simulink model "chris_3R_hsv_mag"  (R2024b)
settings: Solver=FixedStepDiscrete  StartTime=0.0  StopTime=6  FixedStep=0.1  MaxStep=0.1  RelTol=1e-3
libraries: realtime_pacer_lib x1
(part 1 of 2)
settings Model: Creator=RSL  LastModifiedBy=cwaight
settings SolverCC: AlgebraicLoopSolver=TrustRegion
settings DataIOCC: ReturnWorkspaceOutputs=off
settings DebuggingCC: UnconnectedInputMsg=warning  UnconnectedOutputMsg=warning  UnconnectedLineMsg=warning  ArithmeticOperatorsInVariantConditions=warning
settings ModelReferenceCC: EnableRefExpFcnMdlSchedulingChecks=on
settings SFSimCC: SimUseLocalCustomCode=off  CustomCodeUndefinedFunction=UseInterfaceOnly
settings RTWCC: RTWUseLocalCustomCode=off  GPUComputeCapability=3.5
settings CodeAppCC: StateflowObjectComments=on

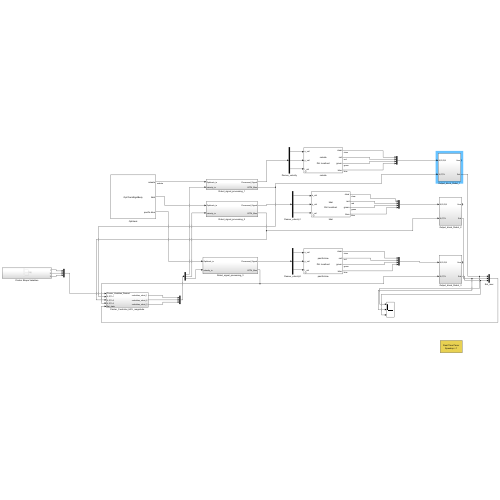
[thumbnail: Simulink's stored preview of the top-level diagram]
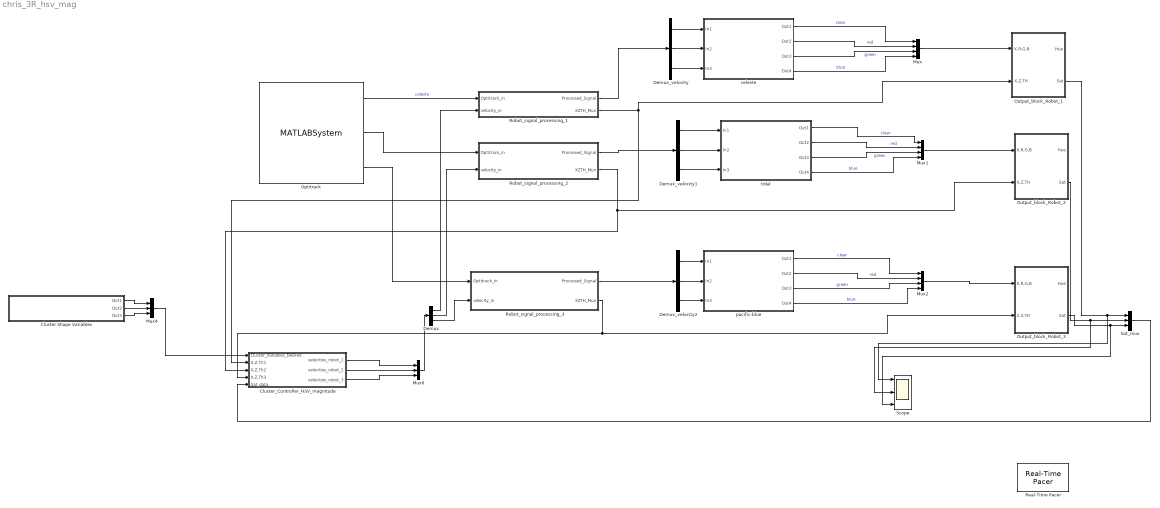
== system chris_3R_hsv_mag ==
  Cluster Shape Variables : Subsystem
  Cluster_Controller_HSV_magnitude : Subsystem
  Demux : Demux  Outputs=3
  Demux_velocity : Demux  Outputs=3
  Demux_velocity1 : Demux  Outputs=3
  Demux_velocity2 : Demux  Outputs=3
  Mux : Mux
  Mux1 : Mux
  Mux2 : Mux
  Mux4 : Mux  Inputs=3
  Mux6 : Mux  Inputs=3
  Optitrack : MATLABSystem  System=OptiTrackRigidBody  coordinateTransformationMatrix=[ 1, 0, 0; 0, 0, 1; 0, -1, 0 ]  rigidBodyNames={ 'celeste','tidal','pacific-blue'}  orientationFormat=Euler angles  debug=on  natNetHostAddress=127.0.0.1  natNetClientAddress=127.0.0.1  dllPath=C:\DecaMATLAB\NatNetSDK\lib\x64\NatNetML.dll  unicast=off
      mask Type: OptiTrackRigidBody
      mask Display:
      | disp('OptiTrackRigidBody');
      | port_label('output',1,'celeste');
      | port_label('output',2,'tidal');
      | port_label('output',3,'pacific-blue');
  Output_block_Robot_1 : Subsystem
  Output_block_Robot_2 : Subsystem
  Output_block_Robot_3 : Subsystem
  Real-Time Pacer : realtime_pacer_lib/Real-Time Pacer  simTimePerRealTime=1
  Robot_signal_processing_1 : Subsystem
  Robot_signal_processing_2 : Subsystem
  Robot_signal_processing_3 : Subsystem
  Sat_mux : Mux  Inputs=3
  Scope : Scope  NumInputPorts=3
  celeste : Subsystem  mask(DecabotMask){robotName=celeste, decabotHelper=localhost, robotAddress=, useDataTurbine=off, useDirectSocket=on, debug=off}
      mask prompts: robotName "Robot name:"; decabotHelper "DecabotHelper/DataTurbine server:"; robotAddress "Robot network address (optional):"; useDataTurbine "Use DataTurbine"; useDirectSocket "Use direct robot TCP connection"; debug "Log debug messages"
      mask help: This is a masked subsystem that contains a Decabot block for bidirectional communication with a decabot over a direct TCP socket connection.
      mask init:
      | robotName = 'Nobody';
      | decabotHelper = 'localhost';
      | robotAddress = '';
      | useDataTurbine = true;
      | debug = true;
      mask TypeOptions robotName: decabot/robotName
      mask Callback robotName:
      | try
      |     set_param( gcb( ), 'Name', get_param( gcb( ), 'robotName' ) );
      | end
      mask TypeOptions decabotHelper: decabot/decabotHelper
      mask TypeOptions robotAddress: decabot/robotAddress
      mask TypeOptions useDataTurbine: decabot/useDataTurbine
      mask TypeOptions useDirectSocket: decabot/useDirectSocket
      mask TypeOptions debug: decabot/debug
      mask Display:
      | disp( [get_param( gcb( ), 'robotName' ) '\n\nDH: ' get_param( gcb( ), 'decabotHelper' ) ] );
      | 
      | port_label('input',1,'x_vel');
      | port_label('input',2,'y_vel');
      | port_label('input',3,'t_vel');
      | 
      | port_label('output',1,'clear');
      | port_label('output',2,'red');
      | port_label('output',3,'green');
      | port_label('output',4,'blue');
  pacific-blue : Subsystem  mask(DecabotMask){robotName=pacific-blue, decabotHelper=localhost, robotAddress=, useDataTurbine=off, useDirectSocket=on, debug=off}
      mask prompts: robotName "Robot name:"; decabotHelper "DecabotHelper/DataTurbine server:"; robotAddress "Robot network address (optional):"; useDataTurbine "Use DataTurbine"; useDirectSocket "Use direct robot TCP connection"; debug "Log debug messages"
      mask help: This is a masked subsystem that contains a Decabot block for bidirectional communication with a decabot over a direct TCP socket connection.
      mask init:
      | robotName = 'Nobody';
      | decabotHelper = 'localhost';
      | robotAddress = '';
      | useDataTurbine = true;
      | debug = true;
      mask TypeOptions robotName: decabot/robotName
      mask Callback robotName:
      | try
      |     set_param( gcb( ), 'Name', get_param( gcb( ), 'robotName' ) );
      | end
      mask TypeOptions decabotHelper: decabot/decabotHelper
      mask TypeOptions robotAddress: decabot/robotAddress
      mask TypeOptions useDataTurbine: decabot/useDataTurbine
      mask TypeOptions useDirectSocket: decabot/useDirectSocket
      mask TypeOptions debug: decabot/debug
      mask Display:
      | disp( [get_param( gcb( ), 'robotName' ) '\n\nDH: ' get_param( gcb( ), 'decabotHelper' ) ] );
      | 
      | port_label('input',1,'x_vel');
      | port_label('input',2,'y_vel');
      | port_label('input',3,'t_vel');
      | 
      | port_label('output',1,'clear');
      | port_label('output',2,'red');
      | port_label('output',3,'green');
      | port_label('output',4,'blue');
  tidal : Subsystem  mask(DecabotMask){robotName=tidal, decabotHelper=localhost, robotAddress=, useDataTurbine=off, useDirectSocket=on, debug=off}
      mask prompts: robotName "Robot name:"; decabotHelper "DecabotHelper/DataTurbine server:"; robotAddress "Robot network address (optional):"; useDataTurbine "Use DataTurbine"; useDirectSocket "Use direct robot TCP connection"; debug "Log debug messages"
      mask help: This is a masked subsystem that contains a Decabot block for bidirectional communication with a decabot over a direct TCP socket connection.
      mask init:
      | robotName = 'Nobody';
      | decabotHelper = 'localhost';
      | robotAddress = '';
      | useDataTurbine = true;
      | debug = true;
      mask TypeOptions robotName: decabot/robotName
      mask Callback robotName:
      | try
      |     set_param( gcb( ), 'Name', get_param( gcb( ), 'robotName' ) );
      | end
      mask TypeOptions decabotHelper: decabot/decabotHelper
      mask TypeOptions robotAddress: decabot/robotAddress
      mask TypeOptions useDataTurbine: decabot/useDataTurbine
      mask TypeOptions useDirectSocket: decabot/useDirectSocket
      mask TypeOptions debug: decabot/debug
      mask Display:
      | disp( [get_param( gcb( ), 'robotName' ) '\n\nDH: ' get_param( gcb( ), 'decabotHelper' ) ] );
      | 
      | port_label('input',1,'x_vel');
      | port_label('input',2,'y_vel');
      | port_label('input',3,'t_vel');
      | 
      | port_label('output',1,'clear');
      | port_label('output',2,'red');
      | port_label('output',3,'green');
      | port_label('output',4,'blue');
  wires:
  Demux_velocity/3 -> celeste/3(In3)
  Demux_velocity/1 -> celeste/1(In1)
  Demux_velocity/2 -> celeste/2(In2)
  Optitrack/1 -> Robot_signal_processing_1/1(Optitrack_in)  "celeste"
  Robot_signal_processing_1/1(Processed_Signal) -> Demux_velocity/1
  celeste/1(Out1) -> Mux/1  "clear"
  celeste/2(Out2) -> Mux/2  "red"
  celeste/3(Out3) -> Mux/3  "green"
  celeste/4(Out4) -> Mux/4  "blue"
  Robot_signal_processing_1/2(XZTH_Mux) -> Output_block_Robot_1/2(X,Z,TH), Cluster_Controller_HSV_magnitude/2(X,Z,Th1)
  Mux/1 -> Output_block_Robot_1/1(K,R,G,B)
  Demux_velocity1/3 -> tidal/3(In3)
  Demux_velocity1/1 -> tidal/1(In1)
  Demux_velocity1/2 -> tidal/2(In2)
  Robot_signal_processing_2/1(Processed_Signal) -> Demux_velocity1/1
  tidal/1(Out1) -> Mux1/1  "clear"
  tidal/2(Out2) -> Mux1/2  "red"
  tidal/3(Out3) -> Mux1/3  "green"
  tidal/4(Out4) -> Mux1/4  "blue"
  Mux1/1 -> Output_block_Robot_2/1(K,R,G,B)
  Demux_velocity2/3 -> pacific-blue/3(In3)
  Demux_velocity2/1 -> pacific-blue/1(In1)
  Demux_velocity2/2 -> pacific-blue/2(In2)
  Robot_signal_processing_3/1(Processed_Signal) -> Demux_velocity2/1
  pacific-blue/1(Out1) -> Mux2/1  "clear"
  pacific-blue/2(Out2) -> Mux2/2  "red"
  pacific-blue/3(Out3) -> Mux2/3  "green"
  pacific-blue/4(Out4) -> Mux2/4  "blue"
  Mux2/1 -> Output_block_Robot_3/1(K,R,G,B)
  Robot_signal_processing_3/2(XZTH_Mux) -> Output_block_Robot_3/2(X,Z,TH), Cluster_Controller_HSV_magnitude/4(X,Z,Th3)
  Optitrack/2 -> Robot_signal_processing_2/1(Optitrack_in)
  Optitrack/3 -> Robot_signal_processing_3/1(Optitrack_in)
  Mux4/1 -> Cluster_Controller_HSV_magnitude/1(Cluster_Variables_Desired)
  Robot_signal_processing_2/2(XZTH_Mux) -> Output_block_Robot_2/2(X,Z,TH), Cluster_Controller_HSV_magnitude/3(X,Z,Th2)
  Cluster Shape Variables/1(Out1) -> Mux4/1
  Cluster Shape Variables/2(Out2) -> Mux4/2
  Cluster Shape Variables/3(Out3) -> Mux4/3
  Demux/1 -> Robot_signal_processing_1/2(velocity_in)
  Demux/2 -> Robot_signal_processing_2/2(velocity_in)
  Demux/3 -> Robot_signal_processing_3/2(velocity_in)
  Mux6/1 -> Demux/1
  Output_block_Robot_1/2(Sat) -> Scope/1, Sat_mux/1
  Output_block_Robot_3/2(Sat) -> Scope/3, Sat_mux/3
  Output_block_Robot_2/2(Sat) -> Scope/2, Sat_mux/2
  Sat_mux/1 -> Cluster_Controller_HSV_magnitude/5(Sat_data)
  Cluster_Controller_HSV_magnitude/1(velocities_robot_1) -> Mux6/1
  Cluster_Controller_HSV_magnitude/2(velocities_robot_2) -> Mux6/2
  Cluster_Controller_HSV_magnitude/3(velocities_robot_3) -> Mux6/3

== system chris_3R_hsv_mag/Cluster Shape Variables ==
  Cluster Variable C : Constant  Value=pi/3
  Cluster_Variable_B : Constant  Value=0.28
  Cluster_variable_A : Constant  Value=0.28
  Out1 : Outport
  Out2 : Outport  Port=2
  Out3 : Outport  Port=3
  wires:
  Cluster_variable_A/1 -> Out1/1
  Cluster Variable C/1 -> Out3/1
  Cluster_Variable_B/1 -> Out2/1

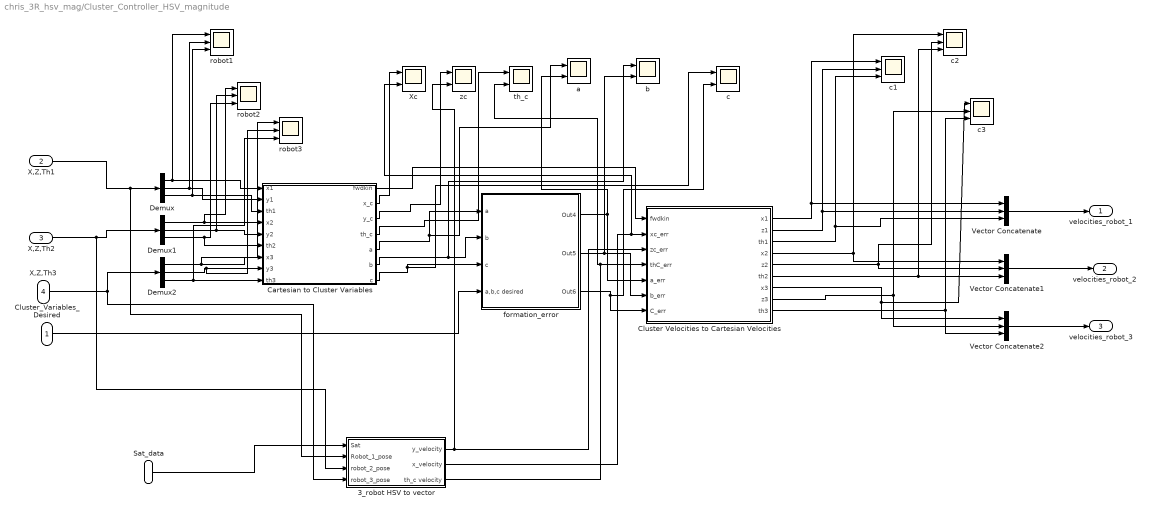
== system chris_3R_hsv_mag/Cluster_Controller_HSV_magnitude ==
  Cluster_Variables_Desired : Inport
  X,Z,Th1 : Inport  Port=2
  X,Z,Th2 : Inport  Port=3
  X,Z,Th3 : Inport  Port=4
  Sat_data : Inport  Port=5
  3_robot HSV to vector : Subsystem
  Cartesian to Cluster Variables : MATLAB Function  TreatAsAtomicUnit=on
  Cluster Velocities to Cartesian Velocities : MATLAB Function  TreatAsAtomicUnit=on
  Demux : Demux  Outputs=3
  Demux1 : Demux  Outputs=3
  Demux2 : Demux  Outputs=3
  Vector Concatenate : Concatenate  NumInputs=3
  Vector Concatenate1 : Concatenate  NumInputs=3
  Vector Concatenate2 : Concatenate  NumInputs=3
  Xc : Scope  NumInputPorts=2
  a : Scope  NumInputPorts=2
  b : Scope  NumInputPorts=2
  c : Scope  NumInputPorts=2
  c1 : Scope  NumInputPorts=3
  c2 : Scope  NumInputPorts=3
  c3 : Scope  NumInputPorts=3
  formation_error : Subsystem
  robot1 : Scope  NumInputPorts=3
  robot2 : Scope  NumInputPorts=3
  robot3 : Scope  NumInputPorts=3
  th_c : Scope  NumInputPorts=2
  zc : Scope  NumInputPorts=2
  velocities_robot_1 : Outport
  velocities_robot_2 : Outport  Port=2
  velocities_robot_3 : Outport  Port=3
  wires:
  X,Z,Th1/1 -> 3_robot HSV to vector/2(Robot_1_pose), Demux/1
  X,Z,Th2/1 -> 3_robot HSV to vector/3(robot_2_pose), Demux1/1
  X,Z,Th3/1 -> Demux2/1, 3_robot HSV to vector/4(robot_3_pose)
  Vector Concatenate/1 -> velocities_robot_1/1
  Cluster Velocities to Cartesian Velocities/2(z1) -> c1/2, Vector Concatenate/2
  Cluster Velocities to Cartesian Velocities/1(x1) -> c1/1, Vector Concatenate/1
  Vector Concatenate1/1 -> velocities_robot_2/1
  Cluster Velocities to Cartesian Velocities/5(z2) -> c2/2, Vector Concatenate1/2
  Cluster Velocities to Cartesian Velocities/4(x2) -> c2/1, Vector Concatenate1/1
  Vector Concatenate2/1 -> velocities_robot_3/1
  Cluster Velocities to Cartesian Velocities/8(z3) -> c3/2, Vector Concatenate2/2
  Cluster Velocities to Cartesian Velocities/7(x3) -> Vector Concatenate2/1, c3/1
  Demux/1 -> robot1/1, Cartesian to Cluster Variables/1(x1)
  Demux/2 -> robot1/2, Cartesian to Cluster Variables/2(y1)
  Demux/3 -> robot1/3, Cartesian to Cluster Variables/3(th1)
  Demux1/1 -> robot2/1, Cartesian to Cluster Variables/4(x2)
  Demux1/2 -> robot2/2, Cartesian to Cluster Variables/5(y2)
  Demux1/3 -> robot2/3, Cartesian to Cluster Variables/6(th2)
  Demux2/1 -> robot3/1, Cartesian to Cluster Variables/7(x3)
  Demux2/2 -> robot3/2, Cartesian to Cluster Variables/8(y3)
  Demux2/3 -> robot3/3, Cartesian to Cluster Variables/9(th3)
  Cartesian to Cluster Variables/2(x_c) -> Xc/1
  Cartesian to Cluster Variables/3(y_c) -> zc/1
  Cartesian to Cluster Variables/4(th_c) -> th_c/1
  Cartesian to Cluster Variables/5(a) -> a/1, formation_error/1(a)
  Cartesian to Cluster Variables/6(b) -> b/1, formation_error/2(b)
  Cartesian to Cluster Variables/7(c) -> c/1, formation_error/3(c)
  Cluster_Variables_Desired/1 -> formation_error/4(a,b,c desired)
  formation_error/1(Out4) -> a/2, Cluster Velocities to Cartesian Velocities/5(a_err)
  formation_error/2(Out5) -> b/2, Cluster Velocities to Cartesian Velocities/6(b_err)
  formation_error/3(Out6) -> Cluster Velocities to Cartesian Velocities/7(C_err), c/2
  Cartesian to Cluster Variables/1(fwdkin) -> Cluster Velocities to Cartesian Velocities/1(fwdkin)
  Cluster Velocities to Cartesian Velocities/3(th1) -> c1/3, Vector Concatenate/3
  Cluster Velocities to Cartesian Velocities/6(th2) -> c2/3, Vector Concatenate1/3
  Cluster Velocities to Cartesian Velocities/9(th3) -> c3/3, Vector Concatenate2/3
  Sat_data/1 -> 3_robot HSV to vector/1(Sat)
  3_robot HSV to vector/2(x_velocity) -> Xc/2, Cluster Velocities to Cartesian Velocities/2(xc_err)
  3_robot HSV to vector/1(y_velocity) -> Cluster Velocities to Cartesian Velocities/3(zc_err), zc/2
  3_robot HSV to vector/3(th_c velocity) -> Cluster Velocities to Cartesian Velocities/4(thC_err), th_c/2

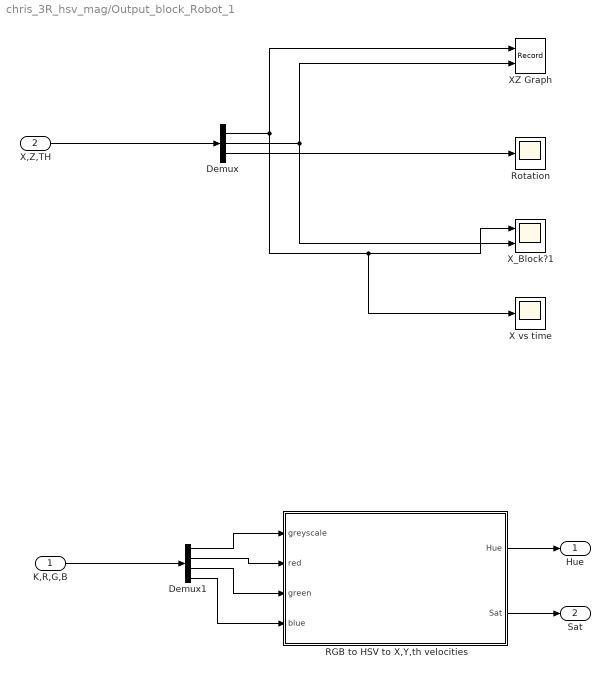
== system chris_3R_hsv_mag/Output_block_Robot_1 ==
  K,R,G,B : Inport
  X,Z,TH : Inport  Port=2
  Demux : Demux  Outputs=3
  Demux1 : Demux
  RGB to HSV to X,Y,th velocities : Subsystem
  Rotation : Scope
  X vs time : Scope
  XZ Graph : Record  FileSettingsInternal="{\"entries\":[{\"content\":{\"excelSettings\":{\"content\":{},\"type\":\"Streamout.ExcelSettings\"}},\"type\":\"Streamout.FileSettingStorage\",\"uuid\":\"\"}],\"packageUris\":[\"http:\\/\\/schema.mathworks.com\\/mf0\\/streamout_blocks\\/R2020a\"],\"version\":\"1.0\"}"  Layout=[1 1]  SignalsInternal="{\"entries\":[{\"content\":{\"signals\":[{\"content\":{\"blockPath\":[],\"dimensions\":[1],\"domain\":\"\",\"lineColor\":\"#fe330a\",\"lineWidth\":2,\"port\":1,\"sid\":[\"\"],\"signalID\":1,\"signalName\":\"Demux:1\"},\"type\":\"RecordBlkView.Signal\",\"uuid\":\"\"},{\"content\":{\"blockPath\":[],\"dimensions\":[1],\"domain\":\"\",\"lineColor\":\"#22b573\",\"lineWidth\":2,\"port\":2,\"sid\":[\"\"],\"signalID\":2,\"signalName\":\"Demux:2\"},\"type\":\"RecordBlkView.Signal\",\"uuid\":\"\"}]},\"type\":\"RecordBlkView.InputSignals\",\"uuid\":\"\"}],\"packageUris\":[\"http:\\/\\/schema.mathworks.com\\/mf0\\/streamout_blocks\\/R2020a\"],\"version\":\"1.0\"}"  VisualizationBindings="{\"xyplotplugin\":{\"info\":[{\"series\":[],\"subplotID\":1}]}}"  CompatibilityTag=XY  st=-1
  X_Block?1 : Scope  NumInputPorts=2
  Hue : Outport
  Sat : Outport  Port=2
  wires:
  Demux/3 -> Rotation/1
  Demux/2 -> X_Block?1/2, XZ Graph/2
  X,Z,TH/1 -> Demux/1
  Demux/1 -> X vs time/1, X_Block?1/1, XZ Graph/1
  K,R,G,B/1 -> Demux1/1
  Demux1/1 -> RGB to HSV to X,Y,th velocities/1(greyscale)
  Demux1/2 -> RGB to HSV to X,Y,th velocities/2(red)
  Demux1/3 -> RGB to HSV to X,Y,th velocities/3(green)
  Demux1/4 -> RGB to HSV to X,Y,th velocities/4(blue)
  RGB to HSV to X,Y,th velocities/1(Hue) -> Hue/1
  RGB to HSV to X,Y,th velocities/2(Sat) -> Sat/1

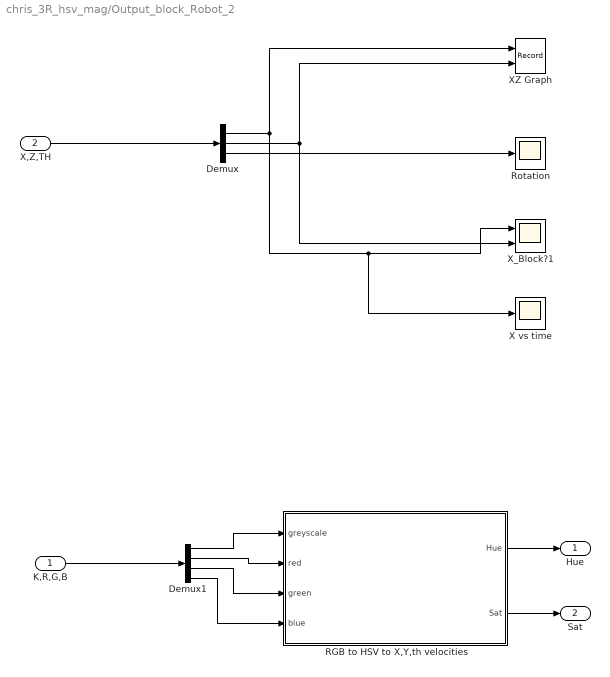
== system chris_3R_hsv_mag/Output_block_Robot_2 ==
  K,R,G,B : Inport
  X,Z,TH : Inport  Port=2
  Demux : Demux  Outputs=3
  Demux1 : Demux
  RGB to HSV to X,Y,th velocities : Subsystem
  Rotation : Scope
  X vs time : Scope
  XZ Graph : Record  FileSettingsInternal="{\"entries\":[{\"content\":{\"excelSettings\":{\"content\":{},\"type\":\"Streamout.ExcelSettings\"}},\"type\":\"Streamout.FileSettingStorage\",\"uuid\":\"\"}],\"packageUris\":[\"http:\\/\\/schema.mathworks.com\\/mf0\\/streamout_blocks\\/R2020a\"],\"version\":\"1.0\"}"  Layout=[1 1]  SignalsInternal="{\"entries\":[{\"content\":{\"signals\":[{\"content\":{\"blockPath\":[],\"dimensions\":[1],\"domain\":\"\",\"lineColor\":\"#edb120\",\"lineWidth\":2,\"port\":1,\"sid\":[\"\"],\"signalID\":1,\"signalName\":\"Demux:1\"},\"type\":\"RecordBlkView.Signal\",\"uuid\":\"\"},{\"content\":{\"blockPath\":[],\"dimensions\":[1],\"domain\":\"\",\"lineColor\":\"#7e2f8e\",\"lineWidth\":2,\"port\":2,\"sid\":[\"\"],\"signalID\":2,\"signalName\":\"Demux:2\"},\"type\":\"RecordBlkView.Signal\",\"uuid\":\"\"}]},\"type\":\"RecordBlkView.InputSignals\",\"uuid\":\"\"}],\"packageUris\":[\"http:\\/\\/schema.mathworks.com\\/mf0\\/streamout_blocks\\/R2020a\"],\"version\":\"1.0\"}"  VisualizationBindings="{\"xyplotplugin\":{\"info\":[{\"series\":[],\"subplotID\":1}]}}"  CompatibilityTag=XY  st=-1
  X_Block?1 : Scope  NumInputPorts=2
  Hue : Outport
  Sat : Outport  Port=2
  wires:
  Demux/3 -> Rotation/1
  Demux/2 -> X_Block?1/2, XZ Graph/2
  X,Z,TH/1 -> Demux/1
  Demux/1 -> X vs time/1, X_Block?1/1, XZ Graph/1
  K,R,G,B/1 -> Demux1/1
  Demux1/1 -> RGB to HSV to X,Y,th velocities/1(greyscale)
  Demux1/2 -> RGB to HSV to X,Y,th velocities/2(red)
  Demux1/3 -> RGB to HSV to X,Y,th velocities/3(green)
  Demux1/4 -> RGB to HSV to X,Y,th velocities/4(blue)
  RGB to HSV to X,Y,th velocities/1(Hue) -> Hue/1
  RGB to HSV to X,Y,th velocities/2(Sat) -> Sat/1

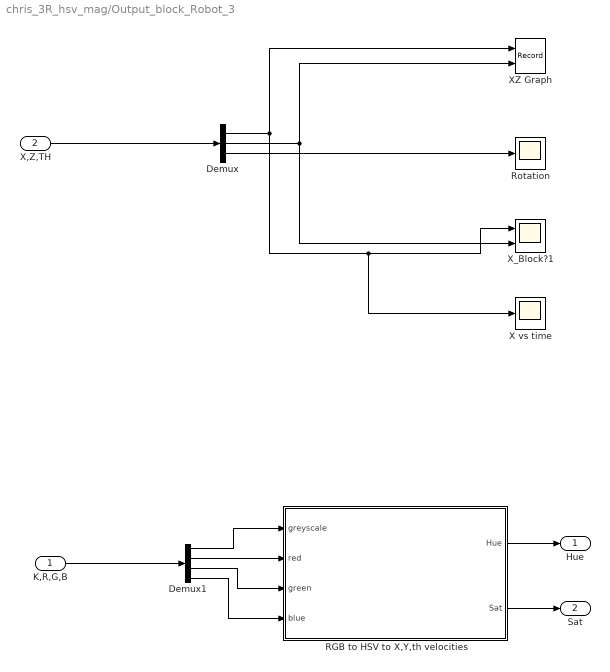
== system chris_3R_hsv_mag/Output_block_Robot_3 ==
  K,R,G,B : Inport
  X,Z,TH : Inport  Port=2
  Demux : Demux  Outputs=3
  Demux1 : Demux
  RGB to HSV to X,Y,th velocities : Subsystem
  Rotation : Scope
  X vs time : Scope
  XZ Graph : Record  FileSettingsInternal="{\"entries\":[{\"content\":{\"excelSettings\":{\"content\":{},\"type\":\"Streamout.ExcelSettings\"}},\"type\":\"Streamout.FileSettingStorage\",\"uuid\":\"\"}],\"packageUris\":[\"http:\\/\\/schema.mathworks.com\\/mf0\\/streamout_blocks\\/R2020a\"],\"version\":\"1.0\"}"  Layout=[1 1]  SignalsInternal="{\"entries\":[{\"content\":{\"signals\":[{\"content\":{\"blockPath\":[],\"dimensions\":[1],\"domain\":\"\",\"lineColor\":\"#a2142f\",\"lineWidth\":2,\"port\":1,\"sid\":[\"\"],\"signalID\":1,\"signalName\":\"Demux:1\"},\"type\":\"RecordBlkView.Signal\",\"uuid\":\"\"},{\"content\":{\"blockPath\":[],\"dimensions\":[1],\"domain\":\"\",\"lineColor\":\"#139fff\",\"lineWidth\":2,\"port\":2,\"sid\":[\"\"],\"signalID\":2,\"signalName\":\"Demux:2\"},\"type\":\"RecordBlkView.Signal\",\"uuid\":\"\"}]},\"type\":\"RecordBlkView.InputSignals\",\"uuid\":\"\"}],\"packageUris\":[\"http:\\/\\/schema.mathworks.com\\/mf0\\/streamout_blocks\\/R2020a\"],\"version\":\"1.0\"}"  VisualizationBindings="{\"xyplotplugin\":{\"info\":[{\"series\":[],\"subplotID\":1}]}}"  CompatibilityTag=XY  st=-1
  X_Block?1 : Scope  NumInputPorts=2
  Hue : Outport
  Sat : Outport  Port=2
  wires:
  Demux/3 -> Rotation/1
  Demux/2 -> X_Block?1/2, XZ Graph/2
  X,Z,TH/1 -> Demux/1
  Demux/1 -> X vs time/1, X_Block?1/1, XZ Graph/1
  K,R,G,B/1 -> Demux1/1
  Demux1/1 -> RGB to HSV to X,Y,th velocities/1(greyscale)
  Demux1/2 -> RGB to HSV to X,Y,th velocities/2(red)
  Demux1/3 -> RGB to HSV to X,Y,th velocities/3(green)
  Demux1/4 -> RGB to HSV to X,Y,th velocities/4(blue)
  RGB to HSV to X,Y,th velocities/1(Hue) -> Hue/1
  RGB to HSV to X,Y,th velocities/2(Sat) -> Sat/1

== system chris_3R_hsv_mag/Robot_signal_processing_1 ==
  Optitrack_in : Inport
  velocity_in : Inport  Port=2
  Demux4 : Demux  Outputs=3
  Global to Body Velocities : Product  Multiplication=Matrix(*)
  Global to Body Rotation Matrix : MATLAB Function  TreatAsAtomicUnit=on
  Math Function : Math  Operator=transpose  SignedPower=on
  Mux : Mux  Inputs=3
  Signal_Reshape : Reshape  OutputDimensions=6
  Signal_Select : Selector  InputPortWidth=6  IndexOptions=Index vector (dialog)  Indices=[1 2 6]  OutputSizes=1
  Processed_Signal : Outport
  XZTH_Mux : Outport  Port=2
  wires:
  Demux4/1 -> Mux/1  "X"
  Demux4/3 -> Mux/3, Global to Body Rotation Matrix/1(u)  "theta"
  Demux4/2 -> Mux/2  "Z"
  Global to Body Velocities/1 -> Processed_Signal/1
  Signal_Reshape/1 -> Signal_Select/1
  velocity_in/1 -> Global to Body Velocities/2
  Optitrack_in/1 -> Signal_Reshape/1
  Global to Body Rotation Matrix/1(y) -> Math Function/1
  Signal_Select/1 -> Demux4/1
  Math Function/1 -> Global to Body Velocities/1
  Mux/1 -> XZTH_Mux/1

== system chris_3R_hsv_mag/Robot_signal_processing_2 ==
  Optitrack_in : Inport
  velocity_in : Inport  Port=2
  Demux4 : Demux  Outputs=3
  Global to Body Velocities : Product  Multiplication=Matrix(*)
  Global to Body Rotation Matrix : MATLAB Function  TreatAsAtomicUnit=on
  Math Function : Math  Operator=transpose  SignedPower=on
  Mux : Mux  Inputs=3
  Signal_Reshape : Reshape  OutputDimensions=6
  Signal_Select : Selector  InputPortWidth=6  IndexOptions=Index vector (dialog)  Indices=[1 2 6]  OutputSizes=1
  Processed_Signal : Outport
  XZTH_Mux : Outport  Port=2
  wires:
  Demux4/1 -> Mux/1  "X"
  Demux4/3 -> Mux/3, Global to Body Rotation Matrix/1(u)  "theta"
  Demux4/2 -> Mux/2  "Z"
  Global to Body Velocities/1 -> Processed_Signal/1
  Signal_Reshape/1 -> Signal_Select/1
  velocity_in/1 -> Global to Body Velocities/2
  Optitrack_in/1 -> Signal_Reshape/1
  Global to Body Rotation Matrix/1(y) -> Math Function/1
  Signal_Select/1 -> Demux4/1
  Math Function/1 -> Global to Body Velocities/1
  Mux/1 -> XZTH_Mux/1

== system chris_3R_hsv_mag/Robot_signal_processing_3 ==
  Optitrack_in : Inport
  velocity_in : Inport  Port=2
  Demux4 : Demux  Outputs=3
  Global to Body Velocities : Product  Multiplication=Matrix(*)
  Global to Body Rotation Matrix : MATLAB Function  TreatAsAtomicUnit=on
  Math Function : Math  Operator=transpose  SignedPower=on
  Mux : Mux  Inputs=3
  Signal_Reshape : Reshape  OutputDimensions=6
  Signal_Select : Selector  InputPortWidth=6  IndexOptions=Index vector (dialog)  Indices=[1 2 6]  OutputSizes=1
  Processed_Signal : Outport
  XZTH_Mux : Outport  Port=2
  wires:
  Demux4/1 -> Mux/1  "X"
  Demux4/3 -> Mux/3, Global to Body Rotation Matrix/1(u)  "theta"
  Demux4/2 -> Mux/2  "Z"
  Global to Body Velocities/1 -> Processed_Signal/1
  Signal_Reshape/1 -> Signal_Select/1
  velocity_in/1 -> Global to Body Velocities/2
  Optitrack_in/1 -> Signal_Reshape/1
  Global to Body Rotation Matrix/1(y) -> Math Function/1
  Signal_Select/1 -> Demux4/1
  Math Function/1 -> Global to Body Velocities/1
  Mux/1 -> XZTH_Mux/1

== system chris_3R_hsv_mag/celeste ==
  In1 : Inport
  In2 : Inport  Port=2
  In3 : Inport  Port=3
  Signal Specification : SignalSpecification  OutDataTypeStr=double  Dimensions=1
  Signal Specification1 : SignalSpecification  OutDataTypeStr=double  Dimensions=1
  Signal Specification2 : SignalSpecification  OutDataTypeStr=double  Dimensions=1
  decabot : MATLABSystem  System=Decabot  robotName=celeste  decabotHelper=localhost  useDataTurbine=off  useDirectSocket=on  debug=off
      mask Type: Decabot
      mask Display:
      | disp('celeste\n\nDH: localhost');
      | port_label('input',1,'x_vel');
      | port_label('input',2,'y_vel');
      | port_label('input',3,'t_vel');
      | port_label('output',1,'clear');
      | port_label('output',2,'red');
      | port_label('output',3,'green');
      | port_label('output',4,'blue');
  Out1 : Outport
  Out2 : Outport  Port=2
  Out3 : Outport  Port=3
  Out4 : Outport  Port=4
  wires:
  Signal Specification2/1 -> decabot/3
  Signal Specification1/1 -> decabot/2
  Signal Specification/1 -> decabot/1
  In2/1 -> Signal Specification1/1
  decabot/4 -> Out4/1
  decabot/1 -> Out1/1
  decabot/3 -> Out3/1
  decabot/2 -> Out2/1
  In1/1 -> Signal Specification/1
  In3/1 -> Signal Specification2/1

== system chris_3R_hsv_mag/pacific-blue ==
  In1 : Inport
  In2 : Inport  Port=2
  In3 : Inport  Port=3
  Signal Specification : SignalSpecification  OutDataTypeStr=double  Dimensions=1
  Signal Specification1 : SignalSpecification  OutDataTypeStr=double  Dimensions=1
  Signal Specification2 : SignalSpecification  OutDataTypeStr=double  Dimensions=1
  decabot : MATLABSystem  System=Decabot  robotName=pacific-blue  decabotHelper=localhost  useDataTurbine=off  useDirectSocket=on  debug=off
      mask Type: Decabot
      mask Display:
      | disp('pacific-blue\n\nDH: localhost');
      | port_label('input',1,'x_vel');
      | port_label('input',2,'y_vel');
      | port_label('input',3,'t_vel');
      | port_label('output',1,'clear');
      | port_label('output',2,'red');
      | port_label('output',3,'green');
      | port_label('output',4,'blue');
  Out1 : Outport
  Out2 : Outport  Port=2
  Out3 : Outport  Port=3
  Out4 : Outport  Port=4
  wires:
  Signal Specification2/1 -> decabot/3
  Signal Specification1/1 -> decabot/2
  Signal Specification/1 -> decabot/1
  In2/1 -> Signal Specification1/1
  decabot/4 -> Out4/1
  decabot/1 -> Out1/1
  decabot/3 -> Out3/1
  decabot/2 -> Out2/1
  In1/1 -> Signal Specification/1
  In3/1 -> Signal Specification2/1

== system chris_3R_hsv_mag/tidal ==
  In1 : Inport
  In2 : Inport  Port=2
  In3 : Inport  Port=3
  Signal Specification : SignalSpecification  OutDataTypeStr=double  Dimensions=1
  Signal Specification1 : SignalSpecification  OutDataTypeStr=double  Dimensions=1
  Signal Specification2 : SignalSpecification  OutDataTypeStr=double  Dimensions=1
  decabot : MATLABSystem  System=Decabot  robotName=tidal  decabotHelper=localhost  useDataTurbine=off  useDirectSocket=on  debug=off
      mask Type: Decabot
      mask Display:
      | disp('tidal\n\nDH: localhost');
      | port_label('input',1,'x_vel');
      | port_label('input',2,'y_vel');
      | port_label('input',3,'t_vel');
      | port_label('output',1,'clear');
      | port_label('output',2,'red');
      | port_label('output',3,'green');
      | port_label('output',4,'blue');
  Out1 : Outport
  Out2 : Outport  Port=2
  Out3 : Outport  Port=3
  Out4 : Outport  Port=4
  wires:
  Signal Specification2/1 -> decabot/3
  Signal Specification1/1 -> decabot/2
  Signal Specification/1 -> decabot/1
  In2/1 -> Signal Specification1/1
  decabot/4 -> Out4/1
  decabot/1 -> Out1/1
  decabot/3 -> Out3/1
  decabot/2 -> Out2/1
  In1/1 -> Signal Specification/1
  In3/1 -> Signal Specification2/1

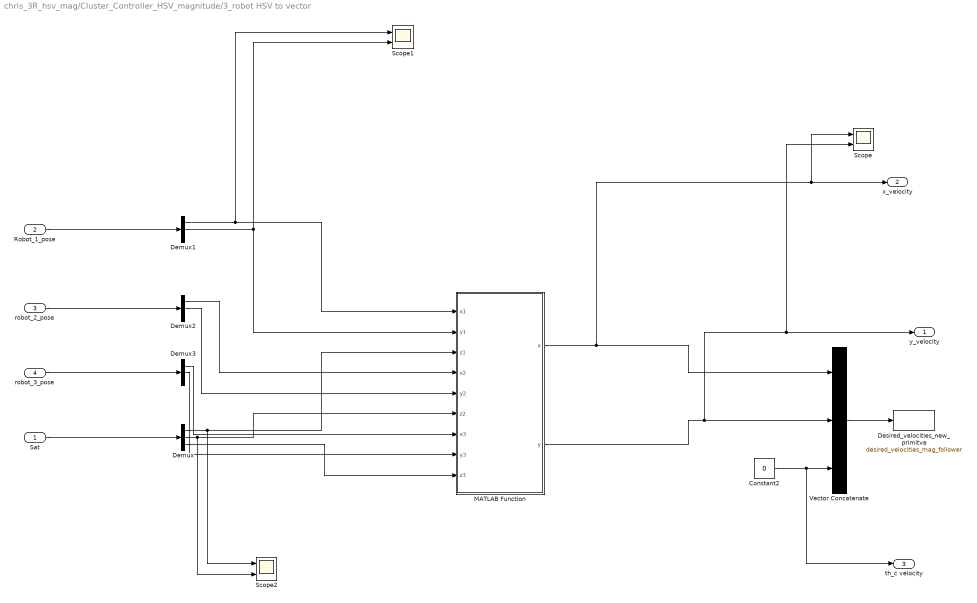
== system chris_3R_hsv_mag/Cluster_Controller_HSV_magnitude/3_robot HSV to vector ==
  Sat : Inport
  Robot_1_pose : Inport  Port=2
  robot_2_pose : Inport  Port=3
  robot_3_pose : Inport  Port=4
  Constant2 : Constant  Value=0
  Demux{,1..3} (4 alike) : Demux  Outputs=3
  Desired_velocities_new_primitve : ToWorkspace  VariableName=desired_velocities_mag_follower  SampleTime=-1
  MATLAB Function : MATLAB Function  TreatAsAtomicUnit=on
  Scope : Scope  NumInputPorts=2
  Scope1 : Scope  NumInputPorts=2
  Scope2 : Scope  NumInputPorts=2
  Vector Concatenate : Concatenate  NumInputs=3
  y_velocity : Outport
  x_velocity : Outport  Port=2
  th_c velocity : Outport  Port=3
  wires:
  Vector Concatenate/1 -> Desired_velocities_new_primitve/1
  Constant2/1 -> th_c velocity/1, Vector Concatenate/3
  Sat/1 -> Demux/1
  Robot_1_pose/1 -> Demux1/1
  robot_2_pose/1 -> Demux2/1
  robot_3_pose/1 -> Demux3/1
  Demux1/1 -> Scope1/1, MATLAB Function/1(x1)
  Demux1/2 -> MATLAB Function/2(y1), Scope1/2
  Demux/1 -> Scope2/1, MATLAB Function/3(z1)
  Demux2/1 -> MATLAB Function/4(x2)
  Demux2/2 -> MATLAB Function/5(y2)
  Demux/2 -> Scope2/2, MATLAB Function/6(z2)
  Demux3/1 -> MATLAB Function/7(x3)
  Demux3/2 -> MATLAB Function/8(y3)
  Demux/3 -> MATLAB Function/9(z3)
  MATLAB Function/1(x) -> Scope/1, x_velocity/1, Vector Concatenate/1
  MATLAB Function/2(y) -> Scope/2, y_velocity/1, Vector Concatenate/2

== system chris_3R_hsv_mag/Cluster_Controller_HSV_magnitude/formation_error ==
  a : Inport
  b : Inport  Port=2
  c : Inport  Port=3
  a,b,c desired : Inport  Port=4
  Demux7 : Demux  Outputs=3
  Sum3 : Sum  Inputs=-+
  Sum4 : Sum  Inputs=-+
  Sum5 : Sum  Inputs=-+
  Out4 : Outport
  Out5 : Outport  Port=2
  Out6 : Outport  Port=3
  wires:
  Sum3/1 -> Out4/1
  Demux7/3 -> Sum5/2
  a,b,c desired/1 -> Demux7/1
  Demux7/1 -> Sum3/2
  b/1 -> Sum4/1
  Demux7/2 -> Sum4/2
  c/1 -> Sum5/1
  Sum4/1 -> Out5/1
  Sum5/1 -> Out6/1
  a/1 -> Sum3/1

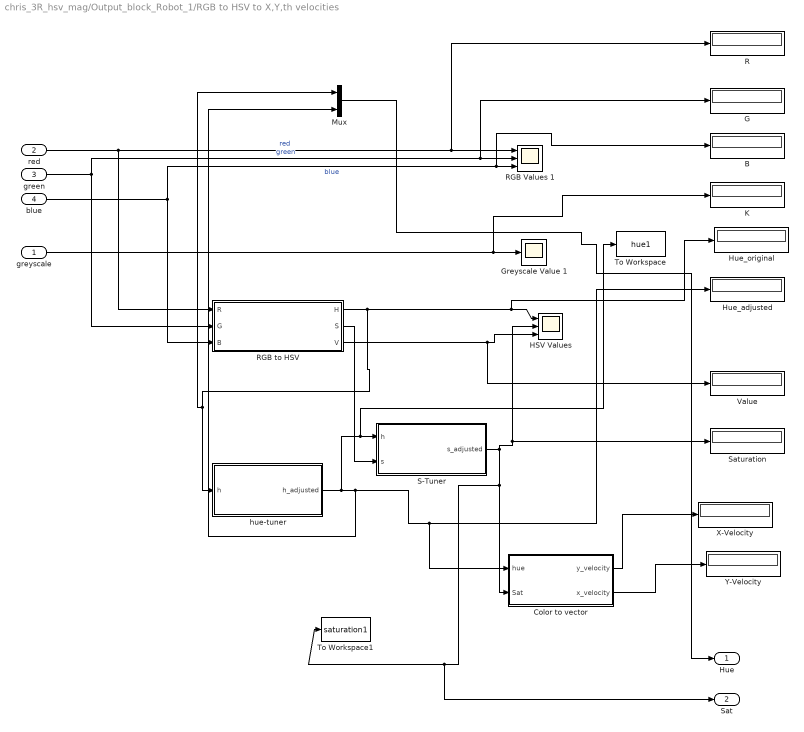
== system chris_3R_hsv_mag/Output_block_Robot_1/RGB to HSV to X,Y,th velocities ==
  greyscale : Inport
  red : Inport  Port=2
  green : Inport  Port=3
  blue : Inport  Port=4
  B : Display
  Color to vector : Subsystem
  G : Display
  Greyscale Value 1 : Scope
  HSV Values : Scope  NumInputPorts=3
  Hue_adjusted : Display
  Hue_original : Display
  K : Display
  Mux : Mux  Inputs=2
  R : Display
  "RGB Values 1 " : Scope  NumInputPorts=3
  RGB to HSV : MATLAB Function  TreatAsAtomicUnit=on
  S-Tuner : MATLAB Function  TreatAsAtomicUnit=on
  Saturation : Display
  To Workspace : ToWorkspace  VariableName=hue1  SaveFormat=Timeseries  SampleTime=-1
  To Workspace1 : ToWorkspace  VariableName=saturation1  SaveFormat=Timeseries  SampleTime=-1
  Value : Display
  X-Velocity : Display
  "Y-Velocity " : Display
  hue-tuner : MATLAB Function  TreatAsAtomicUnit=on
  Hue : Outport
  Sat : Outport  Port=2
  wires:
  red/1 -> R/1, "RGB Values 1 "/1, RGB to HSV/1(R)  "red"
  blue/1 -> B/1, "RGB Values 1 "/3, RGB to HSV/3(B)  "blue"
  greyscale/1 -> K/1, Greyscale Value 1/1
  green/1 -> G/1, "RGB Values 1 "/2, RGB to HSV/2(G)  "green"
  RGB to HSV/3(V) -> Value/1, HSV Values/3
  RGB to HSV/2(S) -> S-Tuner/2(s)
  S-Tuner/1(s_adjusted) -> HSV Values/2, Saturation/1, Sat/1, To Workspace1/1, Color to vector/2(Sat)
  Color to vector/1(y_velocity) -> X-Velocity/1
  Color to vector/2(x_velocity) -> "Y-Velocity "/1
  hue-tuner/1(h_adjusted) -> To Workspace/1, S-Tuner/1(h), Mux/2, Color to vector/1(hue), Hue_adjusted/1
  Mux/1 -> Hue/1
  RGB to HSV/1(H) -> Hue_original/1, HSV Values/1, Mux/1, hue-tuner/1(h)

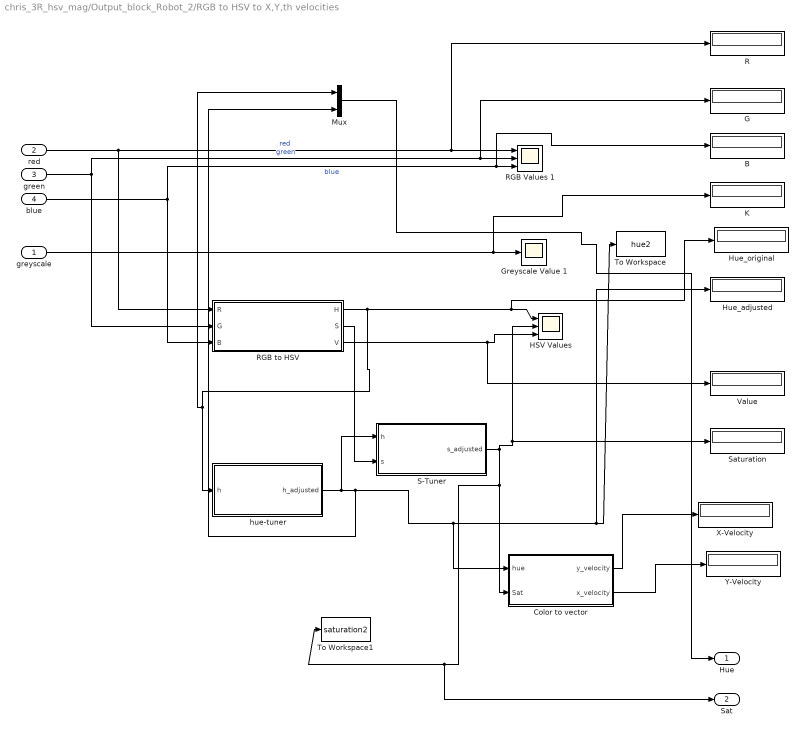
== system chris_3R_hsv_mag/Output_block_Robot_2/RGB to HSV to X,Y,th velocities ==
  greyscale : Inport
  red : Inport  Port=2
  green : Inport  Port=3
  blue : Inport  Port=4
  B : Display
  Color to vector : Subsystem
  G : Display
  Greyscale Value 1 : Scope
  HSV Values : Scope  NumInputPorts=3
  Hue_adjusted : Display
  Hue_original : Display
  K : Display
  Mux : Mux  Inputs=2
  R : Display
  "RGB Values 1 " : Scope  NumInputPorts=3
  RGB to HSV : MATLAB Function  TreatAsAtomicUnit=on
  S-Tuner : MATLAB Function  TreatAsAtomicUnit=on
  Saturation : Display
  To Workspace : ToWorkspace  VariableName=hue2  SaveFormat=Timeseries  SampleTime=-1
  To Workspace1 : ToWorkspace  VariableName=saturation2  SaveFormat=Timeseries  SampleTime=-1
  Value : Display
  X-Velocity : Display
  "Y-Velocity " : Display
  hue-tuner : MATLAB Function  TreatAsAtomicUnit=on
  Hue : Outport
  Sat : Outport  Port=2
  wires:
  red/1 -> R/1, "RGB Values 1 "/1, RGB to HSV/1(R)  "red"
  blue/1 -> B/1, "RGB Values 1 "/3, RGB to HSV/3(B)  "blue"
  greyscale/1 -> K/1, Greyscale Value 1/1
  green/1 -> G/1, "RGB Values 1 "/2, RGB to HSV/2(G)  "green"
  RGB to HSV/3(V) -> Value/1, HSV Values/3
  RGB to HSV/2(S) -> S-Tuner/2(s)
  S-Tuner/1(s_adjusted) -> HSV Values/2, Saturation/1, Sat/1, To Workspace1/1, Color to vector/2(Sat)
  Color to vector/1(y_velocity) -> X-Velocity/1
  Color to vector/2(x_velocity) -> "Y-Velocity "/1
  hue-tuner/1(h_adjusted) -> S-Tuner/1(h), Mux/2, Color to vector/1(hue), To Workspace/1, Hue_adjusted/1
  Mux/1 -> Hue/1
  RGB to HSV/1(H) -> Hue_original/1, HSV Values/1, Mux/1, hue-tuner/1(h)

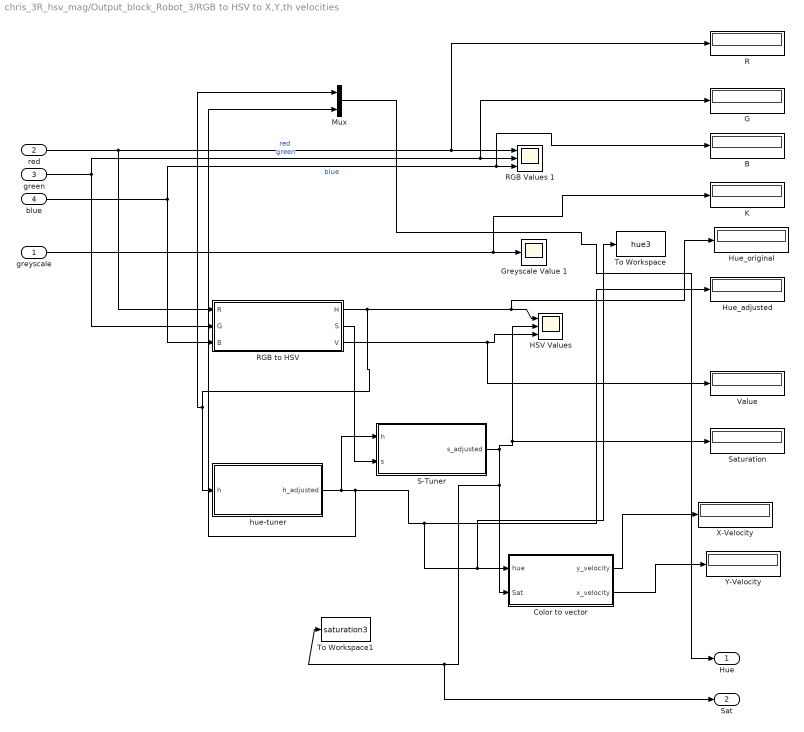
== system chris_3R_hsv_mag/Output_block_Robot_3/RGB to HSV to X,Y,th velocities ==
  greyscale : Inport
  red : Inport  Port=2
  green : Inport  Port=3
  blue : Inport  Port=4
  B : Display
  Color to vector : Subsystem
  G : Display
  Greyscale Value 1 : Scope
  HSV Values : Scope  NumInputPorts=3
  Hue_adjusted : Display
  Hue_original : Display
  K : Display
  Mux : Mux  Inputs=2
  R : Display
  "RGB Values 1 " : Scope  NumInputPorts=3
  RGB to HSV : MATLAB Function  TreatAsAtomicUnit=on
  S-Tuner : MATLAB Function  TreatAsAtomicUnit=on
  Saturation : Display
  To Workspace : ToWorkspace  VariableName=hue3  SaveFormat=Timeseries  SampleTime=-1
  To Workspace1 : ToWorkspace  VariableName=saturation3  SaveFormat=Timeseries  SampleTime=-1
  Value : Display
  X-Velocity : Display
  "Y-Velocity " : Display
  hue-tuner : MATLAB Function  TreatAsAtomicUnit=on
  Hue : Outport
  Sat : Outport  Port=2
  wires:
  red/1 -> R/1, "RGB Values 1 "/1, RGB to HSV/1(R)  "red"
  blue/1 -> B/1, "RGB Values 1 "/3, RGB to HSV/3(B)  "blue"
  greyscale/1 -> K/1, Greyscale Value 1/1
  green/1 -> G/1, "RGB Values 1 "/2, RGB to HSV/2(G)  "green"
  RGB to HSV/3(V) -> Value/1, HSV Values/3
  RGB to HSV/2(S) -> S-Tuner/2(s)
  S-Tuner/1(s_adjusted) -> HSV Values/2, Saturation/1, Sat/1, To Workspace1/1, Color to vector/2(Sat)
  Color to vector/1(y_velocity) -> X-Velocity/1
  Color to vector/2(x_velocity) -> "Y-Velocity "/1
  hue-tuner/1(h_adjusted) -> S-Tuner/1(h), Mux/2, To Workspace/1, Color to vector/1(hue), Hue_adjusted/1
  Mux/1 -> Hue/1
  RGB to HSV/1(H) -> Hue_original/1, HSV Values/1, Mux/1, hue-tuner/1(h)

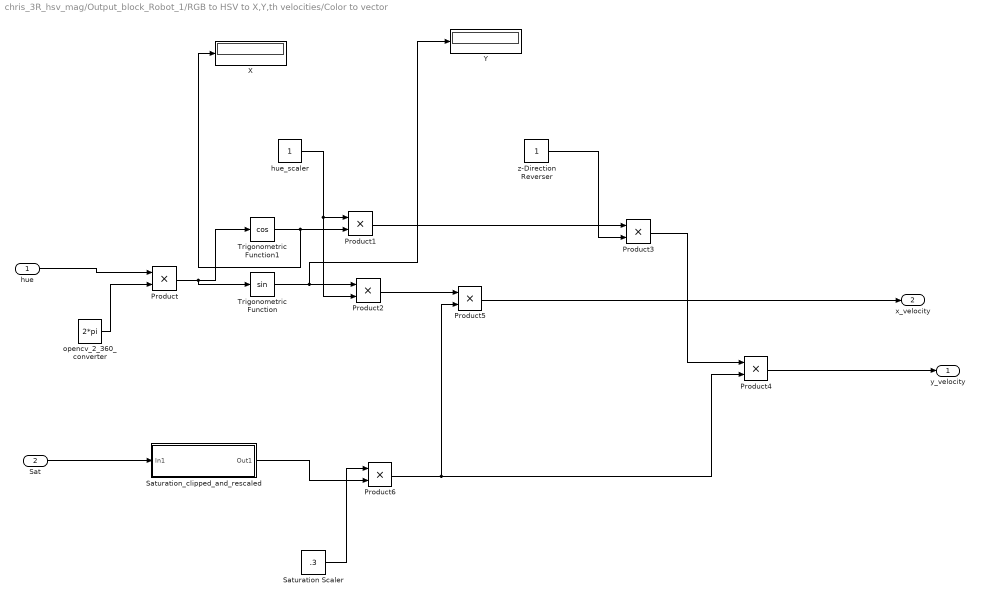
== system chris_3R_hsv_mag/Output_block_Robot_1/RGB to HSV to X,Y,th velocities/Color to vector ==
  hue : Inport
  Sat : Inport  Port=2
  Product{,1..6} (7 alike) : Product
  Saturation Scaler : Constant  Value=.3
  Saturation_clipped_and_rescaled : Subsystem
  Trigonometric Function : Trigonometry
  Trigonometric Function1 : Trigonometry  Operator=cos
  X : Display
  Y : Display
  hue_scaler : Constant
  opencv_2_360_converter : Constant  Value=2*pi
  z-Direction Reverser : Constant
  y_velocity : Outport
  x_velocity : Outport  Port=2
  wires:
  Trigonometric Function/1 -> Y/1, Product2/1
  opencv_2_360_converter/1 -> Product/2
  Product2/1 -> Product5/1
  Trigonometric Function1/1 -> X/1, Product1/2
  Product/1 -> Trigonometric Function1/1, Trigonometric Function/1
  Product1/1 -> Product3/1
  hue/1 -> Product/1
  hue_scaler/1 -> Product2/2, Product1/1
  z-Direction Reverser/1 -> Product3/2
  Product3/1 -> Product4/1
  Product5/1 -> x_velocity/1
  Saturation Scaler/1 -> Product6/1
  Product6/1 -> Product4/2, Product5/2
  Product4/1 -> y_velocity/1
  Sat/1 -> Saturation_clipped_and_rescaled/1(In1)
  Saturation_clipped_and_rescaled/1(Out1) -> Product6/2

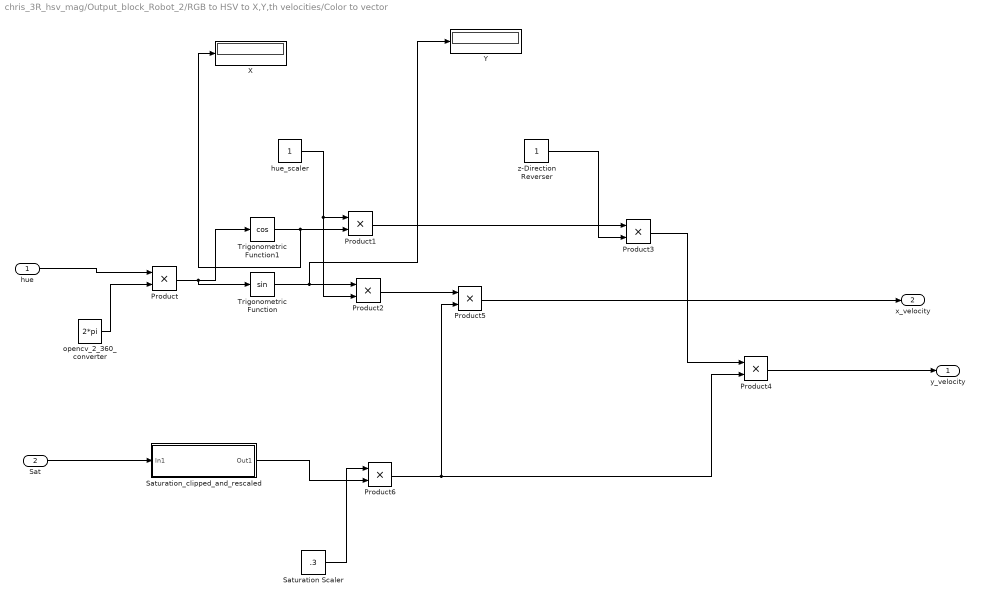
== system chris_3R_hsv_mag/Output_block_Robot_2/RGB to HSV to X,Y,th velocities/Color to vector ==
  hue : Inport
  Sat : Inport  Port=2
  Product{,1..6} (7 alike) : Product
  Saturation Scaler : Constant  Value=.3
  Saturation_clipped_and_rescaled : Subsystem
  Trigonometric Function : Trigonometry
  Trigonometric Function1 : Trigonometry  Operator=cos
  X : Display
  Y : Display
  hue_scaler : Constant
  opencv_2_360_converter : Constant  Value=2*pi
  z-Direction Reverser : Constant
  y_velocity : Outport
  x_velocity : Outport  Port=2
  wires:
  Trigonometric Function/1 -> Y/1, Product2/1
  opencv_2_360_converter/1 -> Product/2
  Product2/1 -> Product5/1
  Trigonometric Function1/1 -> X/1, Product1/2
  Product/1 -> Trigonometric Function1/1, Trigonometric Function/1
  Product1/1 -> Product3/1
  hue/1 -> Product/1
  hue_scaler/1 -> Product2/2, Product1/1
  z-Direction Reverser/1 -> Product3/2
  Product3/1 -> Product4/1
  Product5/1 -> x_velocity/1
  Saturation Scaler/1 -> Product6/1
  Product6/1 -> Product4/2, Product5/2
  Product4/1 -> y_velocity/1
  Sat/1 -> Saturation_clipped_and_rescaled/1(In1)
  Saturation_clipped_and_rescaled/1(Out1) -> Product6/2

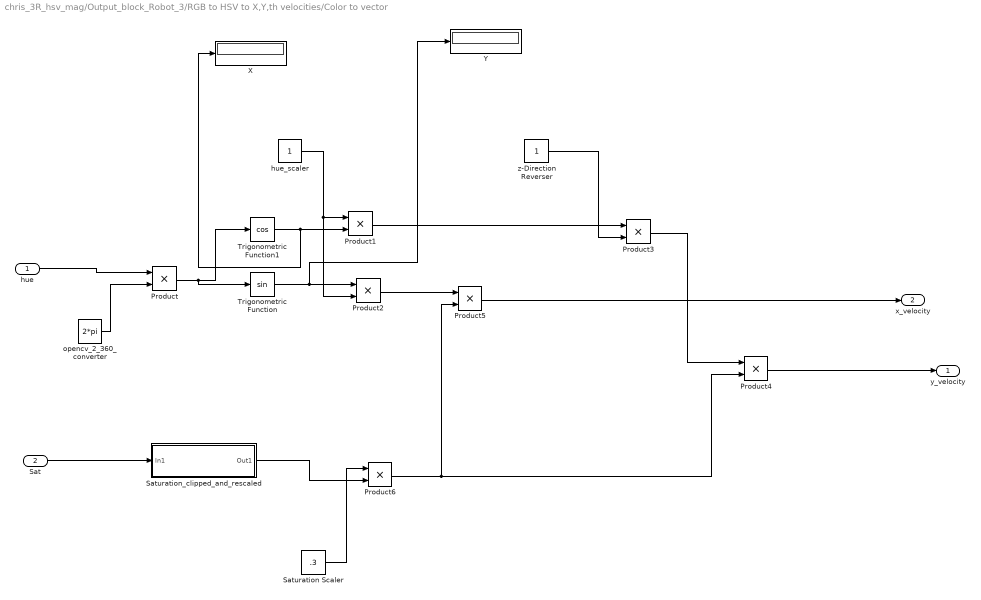
== system chris_3R_hsv_mag/Output_block_Robot_3/RGB to HSV to X,Y,th velocities/Color to vector ==
  hue : Inport
  Sat : Inport  Port=2
  Product{,1..6} (7 alike) : Product
  Saturation Scaler : Constant  Value=.3
  Saturation_clipped_and_rescaled : Subsystem
  Trigonometric Function : Trigonometry
  Trigonometric Function1 : Trigonometry  Operator=cos
  X : Display
  Y : Display
  hue_scaler : Constant
  opencv_2_360_converter : Constant  Value=2*pi
  z-Direction Reverser : Constant
  y_velocity : Outport
  x_velocity : Outport  Port=2
  wires:
  Trigonometric Function/1 -> Y/1, Product2/1
  opencv_2_360_converter/1 -> Product/2
  Product2/1 -> Product5/1
  Trigonometric Function1/1 -> X/1, Product1/2
  Product/1 -> Trigonometric Function1/1, Trigonometric Function/1
  Product1/1 -> Product3/1
  hue/1 -> Product/1
  hue_scaler/1 -> Product2/2, Product1/1
  z-Direction Reverser/1 -> Product3/2
  Product3/1 -> Product4/1
  Product5/1 -> x_velocity/1
  Saturation Scaler/1 -> Product6/1
  Product6/1 -> Product4/2, Product5/2
  Product4/1 -> y_velocity/1
  Sat/1 -> Saturation_clipped_and_rescaled/1(In1)
  Saturation_clipped_and_rescaled/1(Out1) -> Product6/2

== system chris_3R_hsv_mag/Output_block_Robot_1/RGB to HSV to X,Y,th velocities/Color to vector/Saturation_clipped_and_rescaled ==
  In1 : Inport
  Product7 : Product
  Saturation : Saturate  UpperLimit=1  LowerLimit=0.05
  Sum : Sum  Inputs=|+-
  clipped : Constant  Value=0.3
  rescale : Constant  Value=1.42857
  Out1 : Outport
  wires:
  clipped/1 -> Sum/2
  Saturation/1 -> Out1/1
  In1/1 -> Sum/1
  Product7/1 -> Saturation/1
  rescale/1 -> Product7/2
  Sum/1 -> Product7/1

== system chris_3R_hsv_mag/Output_block_Robot_2/RGB to HSV to X,Y,th velocities/Color to vector/Saturation_clipped_and_rescaled ==
  In1 : Inport
  Product7 : Product
  Saturation : Saturate  UpperLimit=1  LowerLimit=0.05
  Sum : Sum  Inputs=|+-
  clipped : Constant  Value=0.3
  rescale : Constant  Value=1.42857
  Out1 : Outport
  wires:
  clipped/1 -> Sum/2
  Saturation/1 -> Out1/1
  In1/1 -> Sum/1
  Product7/1 -> Saturation/1
  rescale/1 -> Product7/2
  Sum/1 -> Product7/1

== system chris_3R_hsv_mag/Output_block_Robot_3/RGB to HSV to X,Y,th velocities/Color to vector/Saturation_clipped_and_rescaled ==
  In1 : Inport
  Product7 : Product
  Saturation : Saturate  UpperLimit=1  LowerLimit=0.05
  Sum : Sum  Inputs=|+-
  clipped : Constant  Value=0.3
  rescale : Constant  Value=1.42857
  Out1 : Outport
  wires:
  clipped/1 -> Sum/2
  Saturation/1 -> Out1/1
  In1/1 -> Sum/1
  Product7/1 -> Saturation/1
  rescale/1 -> Product7/2
  Sum/1 -> Product7/1

== matlab function chris_3R_hsv_mag/Output_block_Robot_3/RGB to HSV to X,Y,th velocities/RGB to HSV ==
  data: R input; H output; G input; B input; S output; V output
function [H, S, V]= rgb2hsv_func(R, G, B)

% This one is tuned for the robot - pink

  % Clip RGB values to be within the range [100, 1200]
  R = max(min(R, 1800), 200);
  G = max(min(G, 2200), 250);
  B = max(min(B, 1900), 250);

  % Normalize RGB to [0, 1]
  R = (R - 200) / (1800-200); 
  G = (G - 250) / (2200-250);
  B = (B - 250) / (1900-250);

  Cmax = max(max(R, G), B);
  Cmin = min(min(R, G), B);
  delta = Cmax - Cmin;

  H = zeros(size(R));
  S = zeros(size(R));
  V = Cmax;

  % Calculate Hue
  ind = find(delta ~= 0); 
  r_ind = find((Cmax == R) & (delta ~= 0));
  g_ind = find((Cmax == G) & (delta ~= 0));
  b_ind = find((Cmax == B) & (delta ~= 0));

  H(r_ind) = 60 * mod((G(r_ind) - B(r_ind)) ./ delta(r_ind), 6);
  H(g_ind) = 60 * (((B(g_ind) - R(g_ind)) ./ delta(g_ind)) + 2);
  H(b_ind) = 60 * (((R(b_ind) - G(b_ind)) ./ delta(b_ind)) + 4);

  H = H / 360;

  % Calculate Saturation
  S(ind) = delta(ind) ./ Cmax(ind);

end

== matlab function chris_3R_hsv_mag/Output_block_Robot_3/RGB to HSV to X,Y,th velocities/S-Tuner ==
  data: h input; s_adjusted output; s input
function s_adjusted   = saturation_adjust(h,s)
    if 0 <= h && h <= 0.05
        s_adjusted = max(0, (s - 0.1114) * (0.7/0.9129) ) + 0.3;
    elseif 0.05 <= h && h <= 0.1
        s_adjusted = max(0, (s - 0.1915) * (0.7/0.665)) + 0.3;
    elseif 0.1 <= h && h <= 0.15
        s_adjusted = max(0, (s - 0.1613) * (0.7/0.6136)) + 0.3;
    elseif 0.15 <= h && h <= 0.2
        s_adjusted = max(0, (s - 0.1096) * (0.7/0.6058)) + 0.3;
    elseif 0.2 <= h && h <= 0.25
        s_adjusted = max(0, (s - 0.0677) * (0.7/0.5851)) + 0.3;
        
    elseif 0.25 <= h && h <= 0.3
        s_adjusted = max(0, (s + 0.1056) * (0.7/0.7955)) + 0.3;
    elseif 0.3 <= h && h <= 0.35
        s_adjusted = max(0, (s + 0.0671) * (0.7/0.644)) + 0.3;
    elseif 0.35 <= h && h <= 0.4
        s_adjusted = max(0, (s - 0.0036) * (0.7/0.3670)) + 0.3;
    elseif 0.4 <= h && h <= 0.45
        s_adjusted = max(0, (s - 0.0768) * (0.7/0.2182)) + 0.3;
    elseif 0.45 <= h && h <= 0.5
        s_adjusted = max(0, (s - 0.0453) * (0.7/0.4158)) + 0.3;

    elseif 0.5 <= h && h <= 0.55
        s_adjusted = max(0, (s - 0.0776) * (0.7/0.4708)) + 0.3;
    elseif 0.55 <= h && h <= 0.6
        s_adjusted = max(0, (s + 0.19) * (0.7/1.1235)) + 0.3;
    elseif 0.6 <= h && h <= 0.65
        s_adjusted = max(0, (s + 0.0663) * (0.7/0.9176)) + 0.3;
    elseif 0.65 <= h && h <= 0.7
        s_adjusted = max(0, (s - 0.0246) * (0.7/0.6231)) + 0.3;
    elseif 0.7 <= h && h <= 0.75
        s_adjusted = max(0, (s - 0.0774) * (0.7/0.5134)) + 0.3;       
        
    elseif 0.75 <= h && h <= 0.8
        s_adjusted = max(0, (s - 0.1307) * (0.7/0.4236)) + 0.3;
    elseif 0.8 <= h && h <= 0.85
        s_adjusted = max(0, (s - 0.2109) * (0.7/0.4814)) + 0.3;
    elseif 0.85 <= h && h <= 0.9
        s_adjusted = max(0, (s - 0.1347) * (0.7/0.7503)) + 0.3;
    elseif 0.9 <= h && h <= 0.95
        s_adjusted = max(0, (s - 0.0922) * (0.7/0.9583)) + 0.3;
    elseif 0.95 <= h && h <= 1
        s_adjusted = max(0, (s - 0.0796) * (0.7/1.0081)) + 0.3;
                
    else
        s_adjusted = s;  
    end
    
    s_adjusted = min(1, s_adjusted);
end

== matlab function chris_3R_hsv_mag/Output_block_Robot_3/RGB to HSV to X,Y,th velocities/hue-tuner ==
  data: h input; h_adjusted output
function h_adjusted   = hue_adjust(h)
    if 0.021 <= h && h <= 0.3
        h_adjusted = max(0, (h + 0.0207) * 1/0.739);
    elseif 0.3 <= h && h <= 0.5
        h_adjusted = max(0, (h + 0.5696) * 1/2.4058);
    elseif 0.5 <= h && h <= 0.7
        h_adjusted = max(0, h - 0.3632) * 1/0.4533 ;
    elseif 0.7 <= h && h <= .85
        h_adjusted = max(0, (h + 0.498) * 1/1.7413) ;
    elseif 0.85 <= h && h <= 1
        h_adjusted = max(0, (h - 0.6648) * 1/0.3342);
    else
        h_adjusted = h;
    end
    
    h_adjusted = min(1, h_adjusted);
end

== matlab function chris_3R_hsv_mag/Cluster_Controller_HSV_magnitude/3_robot HSV to vector/MATLAB Function ==
  data: x output; x1 input; y output; y1 input; z1 input; x2 input; y2 input; z2 input; x3 input; y3 input; z3 input
function [x, y] = steepestDescent(x1, y1, z1, x2, y2, z2, x3, y3, z3)
  % Create vectors AB and AC
  AB = [x2 - x1, y2 - y1, z2 - z1];
  AC = [x3 - x1, y3 - y1, z3 - z1];

  % Calculate the cross product to get the normal vector
  N = cross(-AB, AC);

  % Get the direction of steepest descent (-N)
  descent =-N;

  % Normalize the vector to have unit length in the xy-plane
  magnitude = sqrt(descent(1)^2 + descent(2)^2);
  x = descent(1) / magnitude;
  y = descent(2) / magnitude;
  x = x/8;
  y = y/8;
end

== matlab function chris_3R_hsv_mag/Cluster_Controller_HSV_magnitude/Cartesian to Cluster Variables ==
  data: fwdkin output; x1 input; x_c output; y1 input; th1 input; x2 input; y2 input; th2 input; x3 input; y3 input; th3 input; y_c output; th_c output; a output; b output; c output
function [fwdkin, x_c, y_c, th_c, a, b, c]   = Forward_Kinematics(x1, y1, th1, x2,y2,th2, x3,y3,th3)
% Centre frame
x_c = (x1+x2+x3)/3;
y_c = (y1+y2+y3)/3;
theta_c = atan2((2/3)*x1 - (1/3)*(x2 + x3), (2/3)*y1 - (1/3)*(y2 + y3));
% SAS Properties of triangle
p = sqrt((x1 - x2)^2 + (y1 - y2)^2);
q = sqrt((x3 - x1)^2 + (y1 - y3)^2);
beta = acos((p^2 + q^2 - (x3 - x2)^2 - (y3 - y2)^2) / (2*p*q));
% Rotation vectors
phi1 = th1 + theta_c;
phi2 = th2 + theta_c;
phi3 = th3 + theta_c;
a =p;
b = q;
c = beta;
th_c = theta_c;
fwdkin = [0 0 0 0 0 0];
fwdkin(1) =a;
fwdkin(2) =b;
fwdkin(3) =c;
fwdkin(4) =x_c;
fwdkin(5) =y_c;
fwdkin(6) =th_c;

== matlab function chris_3R_hsv_mag/Cluster_Controller_HSV_magnitude/Cluster Velocities to Cartesian Velocities ==
  data: fwdkin input; xc_err input; x1 output; zc_err input; thC_err input; a_err input; b_err input; C_err input; z1 output; th1 output; x2 output; z2 output; th2 output; x3 output; z3 output; th3 output
function [x1, z1,th1, x2,z2,th2, x3,z3, th3] = InverseJabobian(fwdkin, xc_err, zc_err, thC_err, a_err, b_err, C_err)
%% Unpacking the information from fwd_kin
p = fwdkin(1);
q = fwdkin(2);
beta = fwdkin(3);
xc = fwdkin(4);
yc = fwdkin(5);
theta_c = fwdkin(6);
yc_err = zc_err;
theta_c_err = thC_err;
p_err = a_err;
q_err = b_err;
beta_err = C_err;
%% Inverse Kinematics
  % Calculate x1, y1, and theta1 (Equations 12, 13, and 14)
r = sqrt((q + p*cos(beta))^2 + (p*sin(beta))^2);
  
x1 = xc + (1/3)*r*sin(theta_c);
y1 = yc + (1/3)*r*cos(theta_c);
%theta1 = phi1 - theta_c;
% Calculate x2, y2, and theta2 (Equations 15, 16, and 17)
x2 = xc + (1/3)*r*sin(theta_c) - p*sin(beta/2 + theta_c);
y2 = yc + (1/3)*r*cos(theta_c) - p*cos(beta/2 + theta_c);
%theta2 = phi2 - theta_c;
% Calculate x3, y3, and theta3 (Equations 18, 19, and 20)
x3 = xc + (1/3)*r*sin(theta_c) + q*sin(beta/2 - theta_c);
y3 = yc + (1/3)*r*cos(theta_c) - q*cos(beta/2 - theta_c);
%theta3 = phi3 - theta_c;
%% Now to take the partial derivates
% syms p q beta xc yc theta_c p_err q_err beta_err xc_err yc_err theta_c_err
% 
% % Define the equations
% eqs = [
%   xc + (1/3)*(sqrt((q + p*cos(beta))^2 + (p*sin(beta))^2))*sin(theta_c); % x1
%   yc + (1/3)*(sqrt((q + p*cos(beta))^2 + (p*sin(beta))^2))*cos(theta_c); % y1
%   xc + (1/3)*(sqrt((q + p*cos(beta))^2 + (p*sin(beta))^2))*sin(theta_c) - p*sin(beta/2 + theta_c); % x2
%   yc + (1/3)*(sqrt((q + p*cos(beta))^2 + (p*sin(beta))^2))*cos(theta_c) - p*cos(beta/2 + theta_c); % y2
%   xc + (1/3)*(sqrt((q + p*cos(beta))^2 + (p*sin(beta))^2))*sin(theta_c) + q*sin(beta/2 - theta_c); % x3
%   yc + (1/3)*(sqrt((q + p*cos(beta))^2 + (p*sin(beta))^2))*cos(theta_c) - q*cos(beta/2 - theta_c)  % y3
% ];
% 
% % Define the variables for differentiation
% vars = [p, q, beta, xc, yc, theta_c];
% 
% % Define the errors
% errs = [p_err, q_err, beta_err, xc_err, yc_err, theta_c_err];
% 
% % Initialize an array to store the sums (as symbolic)
% sums = sym(zeros(length(eqs), 1));
% 
% % Loop through equations and variables
% for i = 1:length(eqs)
%   for j = 1:length(vars)
%     derivative = diff(eqs(i), vars(j));
%     sums(i) = sums(i) + derivative * errs(j);
%   end
% end
% 
% % Display the results
% disp(simplify(sums(1)))
% disp(simplify(sums(2)))
% disp(simplify(sums(3)))
% disp(simplify(sums(4)))
% disp(simplify(sums(5)))
% disp(simplify(sums(6)))
%% Now to sum it all up
x1 =(3*xc_err*(p^2 + 2*cos(beta)*p*q + q^2)^(1/2) + p*p_err*sin(theta_c) + q*q_err*sin(theta_c) + p^2*theta_c_err*cos(theta_c) + q^2*theta_c_err*cos(theta_c) + p*q_err*cos(beta)*sin(theta_c) + p_err*q*cos(beta)*sin(theta_c) + 2*p*q*theta_c_err*cos(beta)*cos(theta_c) - beta_err*p*q*sin(beta)*sin(theta_c))/(3*(p^2 + 2*cos(beta)*p*q + q^2)^(1/2));
 
z1 = (3*yc_err*(p^2 + 2*cos(beta)*p*q + q^2)^(1/2) + p*p_err*cos(theta_c) + q*q_err*cos(theta_c) - p^2*theta_c_err*sin(theta_c) - q^2*theta_c_err*sin(theta_c) + p*q_err*cos(beta)*cos(theta_c) + p_err*q*cos(beta)*cos(theta_c) - beta_err*p*q*sin(beta)*cos(theta_c) - 2*p*q*theta_c_err*cos(beta)*sin(theta_c))/(3*(p^2 + 2*cos(beta)*p*q + q^2)^(1/2));
 
x2 = xc_err - p_err*(sin(beta/2 + theta_c) - (sin(theta_c)*(p + q*cos(beta)))/(3*(p^2 + 2*cos(beta)*p*q + q^2)^(1/2))) - beta_err*((p*cos(beta/2 + theta_c))/2 + (p*q*sin(beta)*sin(theta_c))/(3*(p^2 + 2*cos(beta)*p*q + q^2)^(1/2))) + theta_c_err*((cos(theta_c)*(p^2 + 2*cos(beta)*p*q + q^2)^(1/2))/3 - p*cos(beta/2 + theta_c)) + (q_err*sin(theta_c)*(q + p*cos(beta)))/(3*(p^2 + 2*cos(beta)*p*q + q^2)^(1/2));
 
z2 = yc_err - p_err*(cos(beta/2 + theta_c) - (cos(theta_c)*(p + q*cos(beta)))/(3*(p^2 + 2*cos(beta)*p*q + q^2)^(1/2))) + beta_err*((p*sin(beta/2 + theta_c))/2 - (p*q*sin(beta)*cos(theta_c))/(3*(p^2 + 2*cos(beta)*p*q + q^2)^(1/2))) - (theta_c_err*sin(theta_c)*(p^2 + 2*cos(beta)*p*q + q^2)^(1/2))/3 + p*theta_c_err*sin(beta/2 + theta_c) + (q_err*cos(theta_c)*(q + p*cos(beta)))/(3*(p^2 + 2*cos(beta)*p*q + q^2)^(1/2));
 
x3 = xc_err + q_err*(sin(beta/2 - theta_c) + (sin(theta_c)*(q + p*cos(beta)))/(3*(p^2 + 2*cos(beta)*p*q + q^2)^(1/2))) + beta_err*((q*cos(beta/2 - theta_c))/2 - (p*q*sin(beta)*sin(theta_c))/(3*(p^2 + 2*cos(beta)*p*q + q^2)^(1/2))) + (theta_c_err*cos(theta_c)*(p^2 + 2*cos(beta)*p*q + q^2)^(1/2))/3 - q*theta_c_err*cos(beta/2 - theta_c) + (p_err*sin(theta_c)*(p + q*cos(beta)))/(3*(p^2 + 2*cos(beta)*p*q + q^2)^(1/2));
 
z3 = yc_err - theta_c_err*(q*sin(beta/2 - theta_c) + (sin(theta_c)*(p^2 + 2*cos(beta)*p*q + q^2)^(1/2))/3) - q_err*(cos(beta/2 - theta_c) - (cos(theta_c)*(q + p*cos(beta)))/(3*(p^2 + 2*cos(beta)*p*q + q^2)^(1/2))) + beta_err*((q*sin(beta/2 - theta_c))/2 - (p*q*sin(beta)*cos(theta_c))/(3*(p^2 + 2*cos(beta)*p*q + q^2)^(1/2))) + (p_err*cos(theta_c)*(p + q*cos(beta)))/(3*(p^2 + 2*cos(beta)*p*q + q^2)^(1/2));
 
th1 = 0;
th2 = 0;
th3 = 0;

== matlab function chris_3R_hsv_mag/Robot_signal_processing_2/Global to Body Rotation Matrix ==
  data: u input; y output
function y = fcn(u)

y = [cos(u) -sin(u) 0; sin(u) cos(u) 0; 0 0 1];

== matlab function chris_3R_hsv_mag/Robot_signal_processing_3/Global to Body Rotation Matrix ==
  data: u input; y output
function y = fcn(u)

y = [cos(u) -sin(u) 0; sin(u) cos(u) 0; 0 0 1];

== matlab function chris_3R_hsv_mag/Robot_signal_processing_1/Global to Body Rotation Matrix ==
  data: u input; y output
function y = fcn(u)

y = [cos(u) -sin(u) 0; sin(u) cos(u) 0; 0 0 1];
